simulink library "mylib"  (R2020a)
settings: Solver=VariableStepAuto  StartTime=0.0  StopTime=10.0  RelTol=1e-3
undefined symbols (not defined in the file): d_du_max_pu, dir_to_bus1, dir_to_bus_0L, dir_to_bus_2, dir_to_line1, dir_to_line_0L, dir_to_line_2, du_max_pu, du_ph_max_pu, Fi_0, Fi_T_H, Fi_T_L, Fi_T_M, I0_calc_0L, I0_comp_H, I0_comp_L, I0_comp_M, I0_max_0L, I2_max_2, I_diff1, I_diff2, I_diff3, I_diff4, I_diff5, I_diff_to, I_hight_CT1_G, I_hight_CT2_G, I_low_CT1, I_low_CT2, I_max1, I_max2, I_max3, I_max4, I_max5, I_min_sec_CT1, I_min_sec_CT2, I_unb, Iph_max_0L, Iph_max_2, jmp_in_zone, jmp_in_zone_0L, jmp_in_zone_2, K_dop, max_min1, only_K1_0L, only_K1_2, only_K2_0L, only_K2_2, only_K3_0L, only_K3_2, P_ctl_0, PQ_Fi_ctl_0, Q_ctl_0, S_set_0, set, set1, T_fast, T_I_ctl, T_off, T_on ... (+15)
libraries: $bdroot x184, powerlib_meascontrol x97
(part 5 of 14)

== system mylib/339_i_recalc_ph_v1/RS1 ==
  S : Inport
  R : Inport  Port=2
  12 : Logic  AllPortsSameDT=off  OutDataTypeStr=boolean
  13 : Logic  Operator=NOT  AllPortsSameDT=off  OutDataTypeStr=boolean
  14 : Memory
  15 : Logic  Operator=OR  AllPortsSameDT=off  OutDataTypeStr=boolean
  Q : Outport
  wires:
  13/1 -> 12/2
  S/1 -> 15/2
  R/1 -> 13/1
  15/1 -> 12/1
  12/1 -> Q/1, 14/1
  14/1 -> 15/1

== system mylib/339_i_recalc_ph_v1/RS2 ==
  S : Inport
  R : Inport  Port=2
  12 : Logic  AllPortsSameDT=off  OutDataTypeStr=boolean
  13 : Logic  Operator=NOT  AllPortsSameDT=off  OutDataTypeStr=boolean
  14 : Memory
  15 : Logic  Operator=OR  AllPortsSameDT=off  OutDataTypeStr=boolean
  Q : Outport
  wires:
  13/1 -> 12/2
  S/1 -> 15/2
  R/1 -> 13/1
  15/1 -> 12/1
  12/1 -> Q/1, 14/1
  14/1 -> 15/1

== system mylib/339_i_recalc_ph_v1/ratio_hight1 ==
  hight : Inport
  low : Inport  Port=2
  1 : Switch  Criteria=u2 > Threshold
  15 : RelationalOperator  Operator===  OutDataTypeStr=boolean  RndMeth=Nearest
  16 : Product  Inputs=*/  RndMeth=Zero  SaturateOnIntegerOverflow=on
  17 : RelationalOperator  Operator===  OutDataTypeStr=boolean  RndMeth=Nearest
  18 : Logic  Operator=OR  AllPortsSameDT=off  OutDataTypeStr=boolean
  19 : Constant
  20 : Constant  Value=0
  K : Outport
  wires:
  1/1 -> K/1
  low/1 -> 16/2, 17/1
  15/1 -> 18/1
  19/1 -> 1/1
  17/1 -> 18/2
  16/1 -> 1/3
  20/1 -> 15/2, 17/2
  18/1 -> 1/2
  hight/1 -> 16/1, 15/1

== system mylib/339_i_recalc_ph_v1/ratio_hight18 ==
  hight : Inport
  low : Inport  Port=2
  1 : Switch  Criteria=u2 > Threshold
  15 : RelationalOperator  Operator===  OutDataTypeStr=boolean  RndMeth=Nearest
  16 : Product  Inputs=*/  RndMeth=Zero  SaturateOnIntegerOverflow=on
  17 : RelationalOperator  Operator===  OutDataTypeStr=boolean  RndMeth=Nearest
  18 : Logic  Operator=OR  AllPortsSameDT=off  OutDataTypeStr=boolean
  19 : Constant
  20 : Constant  Value=0
  K : Outport
  wires:
  1/1 -> K/1
  low/1 -> 16/2, 17/1
  15/1 -> 18/1
  19/1 -> 1/1
  17/1 -> 18/2
  16/1 -> 1/3
  20/1 -> 15/2, 17/2
  18/1 -> 1/2
  hight/1 -> 16/1, 15/1

== system mylib/342_u_recalc_ph_v1/K_VT_tr ==
  hight : Inport
  low : Inport  Port=2
  1 : Switch  Criteria=u2 > Threshold
  15 : RelationalOperator  Operator===  OutDataTypeStr=boolean  RndMeth=Nearest
  16 : Product  Inputs=*/  RndMeth=Zero  SaturateOnIntegerOverflow=on
  17 : RelationalOperator  Operator===  OutDataTypeStr=boolean  RndMeth=Nearest
  18 : Logic  Operator=OR  AllPortsSameDT=off  OutDataTypeStr=boolean
  19 : Constant
  20 : Constant  Value=0
  K : Outport
  wires:
  1/1 -> K/1
  low/1 -> 16/2, 17/1
  15/1 -> 18/1
  19/1 -> 1/1
  17/1 -> 18/2
  16/1 -> 1/3
  20/1 -> 15/2, 17/2
  18/1 -> 1/2
  hight/1 -> 16/1, 15/1

== system mylib/342_u_recalc_ph_v1/K_VT_zv ==
  hight : Inport
  low : Inport  Port=2
  1 : Switch  Criteria=u2 > Threshold
  15 : RelationalOperator  Operator===  OutDataTypeStr=boolean  RndMeth=Nearest
  16 : Product  Inputs=*/  RndMeth=Zero  SaturateOnIntegerOverflow=on
  17 : RelationalOperator  Operator===  OutDataTypeStr=boolean  RndMeth=Nearest
  18 : Logic  Operator=OR  AllPortsSameDT=off  OutDataTypeStr=boolean
  19 : Constant
  20 : Constant  Value=0
  K : Outport
  wires:
  1/1 -> K/1
  low/1 -> 16/2, 17/1
  15/1 -> 18/1
  19/1 -> 1/1
  17/1 -> 18/2
  16/1 -> 1/3
  20/1 -> 15/2, 17/2
  18/1 -> 1/2
  hight/1 -> 16/1, 15/1

== system mylib/342_u_recalc_ph_v1/module_Ua_zv ==
  Re : Inport
  Im : Inport  Port=2
  1 : Product  Inputs=**
  2 : Sum
  3 : Product  Inputs=**
  4 : Sqrt  SaturateOnIntegerOverflow=on
  Module : Outport
  wires:
  3/1 -> 2/2
  1/1 -> 2/1
  Im/1 -> 3/1, 3/2
  4/1 -> Module/1
  2/1 -> 4/1
  Re/1 -> 1/2, 1/1

== system mylib/342_u_recalc_ph_v1/module_Uab_zv ==
  Re : Inport
  Im : Inport  Port=2
  1 : Product  Inputs=**
  2 : Sum
  3 : Product  Inputs=**
  4 : Sqrt  SaturateOnIntegerOverflow=on
  Module : Outport
  wires:
  3/1 -> 2/2
  1/1 -> 2/1
  Im/1 -> 3/1, 3/2
  4/1 -> Module/1
  2/1 -> 4/1
  Re/1 -> 1/2, 1/1

== system mylib/342_u_recalc_ph_v1/module_Ub_zv ==
  Re : Inport
  Im : Inport  Port=2
  1 : Product  Inputs=**
  2 : Sum
  3 : Product  Inputs=**
  4 : Sqrt  SaturateOnIntegerOverflow=on
  Module : Outport
  wires:
  3/1 -> 2/2
  1/1 -> 2/1
  Im/1 -> 3/1, 3/2
  4/1 -> Module/1
  2/1 -> 4/1
  Re/1 -> 1/2, 1/1

== system mylib/342_u_recalc_ph_v1/module_Ubc_zv ==
  Re : Inport
  Im : Inport  Port=2
  1 : Product  Inputs=**
  2 : Sum
  3 : Product  Inputs=**
  4 : Sqrt  SaturateOnIntegerOverflow=on
  Module : Outport
  wires:
  3/1 -> 2/2
  1/1 -> 2/1
  Im/1 -> 3/1, 3/2
  4/1 -> Module/1
  2/1 -> 4/1
  Re/1 -> 1/2, 1/1

== system mylib/342_u_recalc_ph_v1/module_Uc_zv ==
  Re : Inport
  Im : Inport  Port=2
  1 : Product  Inputs=**
  2 : Sum
  3 : Product  Inputs=**
  4 : Sqrt  SaturateOnIntegerOverflow=on
  Module : Outport
  wires:
  3/1 -> 2/2
  1/1 -> 2/1
  Im/1 -> 3/1, 3/2
  4/1 -> Module/1
  2/1 -> 4/1
  Re/1 -> 1/2, 1/1

== system mylib/342_u_recalc_ph_v1/module_Uca_zv ==
  Re : Inport
  Im : Inport  Port=2
  1 : Product  Inputs=**
  2 : Sum
  3 : Product  Inputs=**
  4 : Sqrt  SaturateOnIntegerOverflow=on
  Module : Outport
  wires:
  3/1 -> 2/2
  1/1 -> 2/1
  Im/1 -> 3/1, 3/2
  4/1 -> Module/1
  2/1 -> 4/1
  Re/1 -> 1/2, 1/1

== system mylib/342_u_recalc_ph_v1/module_Ufk_tr ==
  Re : Inport
  Im : Inport  Port=2
  1 : Product  Inputs=**
  2 : Sum
  3 : Product  Inputs=**
  4 : Sqrt  SaturateOnIntegerOverflow=on
  Module : Outport
  wires:
  3/1 -> 2/2
  1/1 -> 2/1
  Im/1 -> 3/1, 3/2
  4/1 -> Module/1
  2/1 -> 4/1
  Re/1 -> 1/2, 1/1

== system mylib/342_u_recalc_ph_v1/module_Uhk_tr ==
  Re : Inport
  Im : Inport  Port=2
  1 : Product  Inputs=**
  2 : Sum
  3 : Product  Inputs=**
  4 : Sqrt  SaturateOnIntegerOverflow=on
  Module : Outport
  wires:
  3/1 -> 2/2
  1/1 -> 2/1
  Im/1 -> 3/1, 3/2
  4/1 -> Module/1
  2/1 -> 4/1
  Re/1 -> 1/2, 1/1

== system mylib/342_u_recalc_ph_v1/module_Uhu_tr ==
  Re : Inport
  Im : Inport  Port=2
  1 : Product  Inputs=**
  2 : Sum
  3 : Product  Inputs=**
  4 : Sqrt  SaturateOnIntegerOverflow=on
  Module : Outport
  wires:
  3/1 -> 2/2
  1/1 -> 2/1
  Im/1 -> 3/1, 3/2
  4/1 -> Module/1
  2/1 -> 4/1
  Re/1 -> 1/2, 1/1

== system mylib/342_u_recalc_ph_v1/module_Uuf_tr ==
  Re : Inport
  Im : Inport  Port=2
  1 : Product  Inputs=**
  2 : Sum
  3 : Product  Inputs=**
  4 : Sqrt  SaturateOnIntegerOverflow=on
  Module : Outport
  wires:
  3/1 -> 2/2
  1/1 -> 2/1
  Im/1 -> 3/1, 3/2
  4/1 -> Module/1
  2/1 -> 4/1
  Re/1 -> 1/2, 1/1

== system mylib/Inverse time-delay/ANSI Inverse time-delay ==
  I : Inport
  ANSI_N : Inport  Port=2
  Au_ANSI : Inport  Port=3
  Bu_ANSI : Inport  Port=4
  Cu_ANSI : Inport  Port=5
  Ip : Inport  Port=6
  D : Inport  Port=7
  Constant1 : Constant  Value=6
  Constant2 : Constant  Value=7
  Constant20 : Constant
  Constant21 : Constant  Value=2
  Constant22 : Constant  Value=3
  Constant23 : Constant  Value=4
  Constant25 : Constant  Value=5
  Constant3 : Constant  Value=0
  Constant4 : Constant  Value=8
  Equation ANSI : Subsystem
  Relational Operator{,1..7} (8 alike) : RelationalOperator  Operator===  OutDataTypeStr=boolean  RndMeth=Simplest
  Сoefficient_1 : Subsystem
  Сoefficient_2 : Subsystem
  Сoefficient_3 : Subsystem
  Сoefficient_4 : Subsystem
  Сoefficient_5 : Subsystem
  Сoefficient_6 : Subsystem
  Сoefficient_7 : Subsystem
  Сoefficient_8 User : Subsystem
  td : Outport
  wires:
  Relational Operator/1 -> Сoefficient_1/4(N)
  Constant25/1 -> Relational Operator5/2
  Constant22/1 -> Relational Operator2/2
  Constant3/1 -> Сoefficient_1/3(C_in), Сoefficient_1/2(B_in), Сoefficient_1/1(A_in)
  ANSI_N/1 -> Relational Operator1/1, Relational Operator2/1, Relational Operator7/1, Relational Operator6/1, Relational Operator4/1, Relational Operator5/1, Relational Operator3/1, Relational Operator/1
  Constant23/1 -> Relational Operator3/2
  D/1 -> Equation ANSI/6(D)
  Constant21/1 -> Relational Operator1/2
  Constant20/1 -> Relational Operator/2
  I/1 -> Equation ANSI/2(I)
  Ip/1 -> Equation ANSI/3(Ip)
  Equation ANSI/1(td) -> td/1
  Сoefficient_1/1(A_out) -> Сoefficient_2/1(A_in)
  Сoefficient_1/2(B_out) -> Сoefficient_2/2(B_in)
  Сoefficient_1/3(C_out) -> Сoefficient_2/3(C_in)
  Relational Operator1/1 -> Сoefficient_2/4(N)
  Сoefficient_2/1(A_out) -> Сoefficient_3/1(A_in)
  Сoefficient_2/2(B_out) -> Сoefficient_3/2(B_in)
  Сoefficient_2/3(C_out) -> Сoefficient_3/3(C_in)
  Relational Operator2/1 -> Сoefficient_3/4(N)
  Сoefficient_3/1(A_out) -> Сoefficient_4/1(A_in)
  Сoefficient_3/2(B_out) -> Сoefficient_4/2(B_in)
  Сoefficient_3/3(C_out) -> Сoefficient_4/3(C_in)
  Relational Operator3/1 -> Сoefficient_4/4(N)
  Сoefficient_4/1(A_out) -> Сoefficient_5/1(A_in)
  Сoefficient_4/2(B_out) -> Сoefficient_5/2(B_in)
  Сoefficient_4/3(C_out) -> Сoefficient_5/3(C_in)
  Relational Operator5/1 -> Сoefficient_5/4(N)
  Сoefficient_8 User/1(B_out) -> Equation ANSI/1(B)
  Сoefficient_8 User/2(A_out) -> Equation ANSI/4(A)
  Сoefficient_8 User/3(C_out) -> Equation ANSI/5(C)
  Au_ANSI/1 -> Сoefficient_8 User/5(Au)
  Bu_ANSI/1 -> Сoefficient_8 User/6(Bu)
  Cu_ANSI/1 -> Сoefficient_8 User/7(Cu)
  Сoefficient_5/1(A_out) -> Сoefficient_6/1(A_in)
  Сoefficient_5/2(B_out) -> Сoefficient_6/2(B_in)
  Сoefficient_5/3(C_out) -> Сoefficient_6/3(C_in)
  Constant4/1 -> Relational Operator7/2
  Constant2/1 -> Relational Operator6/2
  Constant1/1 -> Relational Operator4/2
  Relational Operator7/1 -> Сoefficient_8 User/4(N)
  Сoefficient_6/1(A_out) -> Сoefficient_7/1(A_in)
  Сoefficient_6/2(B_out) -> Сoefficient_7/2(B_in)
  Сoefficient_6/3(C_out) -> Сoefficient_7/3(C_in)
  Relational Operator6/1 -> Сoefficient_7/4(N)
  Relational Operator4/1 -> Сoefficient_6/4(N)
  Сoefficient_7/3(C_out) -> Сoefficient_8 User/3(C_in)
  Сoefficient_7/2(B_out) -> Сoefficient_8 User/2(B_in)
  Сoefficient_7/1(A_out) -> Сoefficient_8 User/1(A_in)

== system mylib/Inverse time-delay/ANSI Inverse time-delay inductive disk relay ==
  I : Inport
  ANSI_N_idr : Inport  Port=2
  Au_ANSI_idr : Inport  Port=3
  Bu_ANSI_idr : Inport  Port=4
  Cu_ANSI_idr : Inport  Port=5
  Ip : Inport  Port=6
  D : Inport  Port=7
  Constant1 : Constant  Value=6
  Constant2 : Constant  Value=7
  Constant20 : Constant
  Constant21 : Constant  Value=2
  Constant22 : Constant  Value=3
  Constant23 : Constant  Value=4
  Constant25 : Constant  Value=5
  Constant3 : Constant  Value=0
  Constant4 : Constant  Value=8
  Equation ANSI_idr : Subsystem
  Relational Operator{,1..7} (8 alike) : RelationalOperator  Operator===  OutDataTypeStr=boolean  RndMeth=Simplest
  Сoefficient_1 : Subsystem
  Сoefficient_2 : Subsystem
  Сoefficient_3 : Subsystem
  Сoefficient_4 : Subsystem
  Сoefficient_5 : Subsystem
  Сoefficient_6 : Subsystem
  Сoefficient_7 : Subsystem
  Сoefficient_8 User : Subsystem
  td : Outport
  wires:
  Relational Operator/1 -> Сoefficient_1/4(N)
  Constant25/1 -> Relational Operator5/2
  Constant22/1 -> Relational Operator2/2
  Constant3/1 -> Сoefficient_1/3(C_in), Сoefficient_1/2(B_in), Сoefficient_1/1(A_in)
  ANSI_N_idr/1 -> Relational Operator1/1, Relational Operator2/1, Relational Operator7/1, Relational Operator6/1, Relational Operator4/1, Relational Operator5/1, Relational Operator3/1, Relational Operator/1
  Constant23/1 -> Relational Operator3/2
  D/1 -> Equation ANSI_idr/6(D)
  Constant21/1 -> Relational Operator1/2
  Constant20/1 -> Relational Operator/2
  I/1 -> Equation ANSI_idr/2(I)
  Ip/1 -> Equation ANSI_idr/3(Ip)
  Equation ANSI_idr/1(td) -> td/1
  Сoefficient_1/1(A_out) -> Сoefficient_2/1(A_in)
  Сoefficient_1/2(B_out) -> Сoefficient_2/2(B_in)
  Сoefficient_1/3(C_out) -> Сoefficient_2/3(C_in)
  Relational Operator1/1 -> Сoefficient_2/4(N)
  Сoefficient_2/1(A_out) -> Сoefficient_3/1(A_in)
  Сoefficient_2/2(B_out) -> Сoefficient_3/2(B_in)
  Сoefficient_2/3(C_out) -> Сoefficient_3/3(C_in)
  Relational Operator2/1 -> Сoefficient_3/4(N)
  Сoefficient_3/1(A_out) -> Сoefficient_4/1(A_in)
  Сoefficient_3/2(B_out) -> Сoefficient_4/2(B_in)
  Сoefficient_3/3(C_out) -> Сoefficient_4/3(C_in)
  Relational Operator3/1 -> Сoefficient_4/4(N)
  Сoefficient_4/1(A_out) -> Сoefficient_5/1(A_in)
  Сoefficient_4/2(B_out) -> Сoefficient_5/2(B_in)
  Сoefficient_4/3(C_out) -> Сoefficient_5/3(C_in)
  Relational Operator5/1 -> Сoefficient_5/4(N)
  Сoefficient_8 User/1(B_out) -> Equation ANSI_idr/1(B)
  Сoefficient_8 User/2(A_out) -> Equation ANSI_idr/4(A)
  Сoefficient_8 User/3(C_out) -> Equation ANSI_idr/5(C)
  Au_ANSI_idr/1 -> Сoefficient_8 User/5(Au)
  Bu_ANSI_idr/1 -> Сoefficient_8 User/6(Bu)
  Cu_ANSI_idr/1 -> Сoefficient_8 User/7(Cu)
  Сoefficient_5/1(A_out) -> Сoefficient_6/1(A_in)
  Сoefficient_5/2(B_out) -> Сoefficient_6/2(B_in)
  Сoefficient_5/3(C_out) -> Сoefficient_6/3(C_in)
  Constant4/1 -> Relational Operator7/2
  Constant2/1 -> Relational Operator6/2
  Constant1/1 -> Relational Operator4/2
  Relational Operator7/1 -> Сoefficient_8 User/4(N)
  Сoefficient_6/1(A_out) -> Сoefficient_7/1(A_in)
  Сoefficient_6/2(B_out) -> Сoefficient_7/2(B_in)
  Сoefficient_6/3(C_out) -> Сoefficient_7/3(C_in)
  Relational Operator6/1 -> Сoefficient_7/4(N)
  Relational Operator4/1 -> Сoefficient_6/4(N)
  Сoefficient_7/3(C_out) -> Сoefficient_8 User/3(C_in)
  Сoefficient_7/2(B_out) -> Сoefficient_8 User/2(B_in)
  Сoefficient_7/1(A_out) -> Сoefficient_8 User/1(A_in)

== system mylib/Inverse time-delay/IEC Inverse time-delay ==
  I : Inport
  IEC_N : Inport  Port=2
  ku_IEC : Inport  Port=3
  au_IEC : Inport  Port=4
  Ip : Inport  Port=5
  Tb : Inport  Port=6
  Constant20 : Constant
  Constant21 : Constant  Value=2
  Constant22 : Constant  Value=3
  Constant23 : Constant  Value=4
  Constant25 : Constant  Value=5
  Constant3 : Constant  Value=0
  Equation IEC : Subsystem
  Relational Operator{,1..3,5} (5 alike) : RelationalOperator  Operator===  OutDataTypeStr=boolean  RndMeth=Simplest
  Сoefficient_1 : Subsystem
  Сoefficient_2 : Subsystem
  Сoefficient_3 : Subsystem
  Сoefficient_4 : Subsystem
  Сoefficient_5 User : Subsystem
  td : Outport
  wires:
  Сoefficient_5 User/1(k_out) -> Equation IEC/1(k)
  Сoefficient_1/1(k_out) -> Сoefficient_2/1(k_in)
  Relational Operator/1 -> Сoefficient_1/3(N)
  Relational Operator3/1 -> Сoefficient_4/3(N)
  Constant25/1 -> Relational Operator5/2
  Constant22/1 -> Relational Operator2/2
  Constant3/1 -> Сoefficient_1/2(a_in), Сoefficient_1/1(k_in)
  Relational Operator2/1 -> Сoefficient_3/3(N)
  IEC_N/1 -> Relational Operator1/1, Relational Operator2/1, Relational Operator5/1, Relational Operator3/1, Relational Operator/1
  Constant23/1 -> Relational Operator3/2
  Сoefficient_5 User/2(a_out) -> Equation IEC/3(a)
  Tb/1 -> Equation IEC/5(Tb)
  Relational Operator1/1 -> Сoefficient_2/3(N)
  Constant21/1 -> Relational Operator1/2
  Constant20/1 -> Relational Operator/2
  I/1 -> Equation IEC/2(I)
  Сoefficient_1/2(a_out) -> Сoefficient_2/2(a_in)
  Relational Operator5/1 -> Сoefficient_5 User/3(N)
  Ip/1 -> Equation IEC/4(Ip)
  Equation IEC/1(td) -> td/1
  ku_IEC/1 -> Сoefficient_5 User/4(k_u)
  au_IEC/1 -> Сoefficient_5 User/5(a_u)
  Сoefficient_2/2(a_out) -> Сoefficient_3/2(a_in)
  Сoefficient_2/1(k_out) -> Сoefficient_3/1(k_in)
  Сoefficient_3/1(k_out) -> Сoefficient_4/1(k_in)
  Сoefficient_3/2(a_out) -> Сoefficient_4/2(a_in)
  Сoefficient_4/1(k_out) -> Сoefficient_5 User/1(k)
  Сoefficient_4/2(a_out) -> Сoefficient_5 User/2(a)

== system mylib/Inverse time-delay/IEC Inverse time-delay inductive disk relay ==
  I : Inport
  IEC_N_idr : Inport  Port=2
  ku_IEC_idr : Inport  Port=3
  au_IEC_idr : Inport  Port=4
  Ip : Inport  Port=5
  Tb : Inport  Port=6
  Constant20 : Constant
  Constant21 : Constant  Value=2
  Constant22 : Constant  Value=3
  Constant23 : Constant  Value=4
  Constant25 : Constant  Value=5
  Constant3 : Constant  Value=0
  Equation IEC_idr : Subsystem
  Relational Operator{,1..3,5} (5 alike) : RelationalOperator  Operator===  OutDataTypeStr=boolean  RndMeth=Simplest
  Сoefficient_1 : Subsystem
  Сoefficient_2 : Subsystem
  Сoefficient_3 : Subsystem
  Сoefficient_4 : Subsystem
  Сoefficient_5 User : Subsystem
  td : Outport
  wires:
  Сoefficient_5 User/1(k_out) -> Equation IEC_idr/1(k)
  Сoefficient_1/1(k_out) -> Сoefficient_2/1(k_in)
  Relational Operator/1 -> Сoefficient_1/3(N)
  Relational Operator3/1 -> Сoefficient_4/3(N)
  Constant25/1 -> Relational Operator5/2
  Constant22/1 -> Relational Operator2/2
  Constant3/1 -> Сoefficient_1/2(a_in), Сoefficient_1/1(k_in)
  Сoefficient_4/2(a_out) -> Сoefficient_5 User/2(a)
  Relational Operator2/1 -> Сoefficient_3/3(N)
  IEC_N_idr/1 -> Relational Operator1/1, Relational Operator2/1, Relational Operator5/1, Relational Operator3/1, Relational Operator/1
  Constant23/1 -> Relational Operator3/2
  Сoefficient_4/1(k_out) -> Сoefficient_5 User/1(k)
  Сoefficient_5 User/2(a_out) -> Equation IEC_idr/3(a)
  Tb/1 -> Equation IEC_idr/5(Tb)
  Relational Operator1/1 -> Сoefficient_2/3(N)
  Constant21/1 -> Relational Operator1/2
  Constant20/1 -> Relational Operator/2
  I/1 -> Equation IEC_idr/2(I)
  Сoefficient_1/2(a_out) -> Сoefficient_2/2(a_in)
  Relational Operator5/1 -> Сoefficient_5 User/3(N)
  Ip/1 -> Equation IEC_idr/4(Ip)
  Equation IEC_idr/1(td) -> td/1
  ku_IEC_idr/1 -> Сoefficient_5 User/4(k_u)
  au_IEC_idr/1 -> Сoefficient_5 User/5(a_u)
  Сoefficient_2/2(a_out) -> Сoefficient_3/2(a_in)
  Сoefficient_2/1(k_out) -> Сoefficient_3/1(k_in)
  Сoefficient_3/1(k_out) -> Сoefficient_4/1(k_in)
  Сoefficient_3/2(a_out) -> Сoefficient_4/2(a_in)

== system mylib/derivative/fifo2 ==
  y : Inport
  {1..7} (7 alike) : Memory
  y0 : Outport
  y1 : Outport  Port=2
  y2 : Outport  Port=3
  y3 : Outport  Port=4
  y4 : Outport  Port=5
  y5 : Outport  Port=6
  y6 : Outport  Port=7
  y7 : Outport  Port=8
  wires:
  y/1 -> y0/1, 1/1
  1/1 -> y1/1, 2/1
  2/1 -> 3/1, y2/1
  3/1 -> 4/1, y3/1
  4/1 -> 5/1, y4/1
  5/1 -> 6/1, y5/1
  6/1 -> 7/1, y6/1
  7/1 -> y7/1

== system mylib/relative/fifo1 ==
  y : Inport
  {1..7} (7 alike) : Memory
  y0 : Outport
  y1 : Outport  Port=2
  y2 : Outport  Port=3
  y3 : Outport  Port=4
  y4 : Outport  Port=5
  y5 : Outport  Port=6
  y6 : Outport  Port=7
  y7 : Outport  Port=8
  wires:
  y/1 -> y0/1, 1/1
  1/1 -> y1/1, 2/1
  2/1 -> 3/1, y2/1
  3/1 -> 4/1, y3/1
  4/1 -> 5/1, y4/1
  5/1 -> 6/1, y5/1
  6/1 -> 7/1, y6/1
  7/1 -> y7/1

== system mylib/relative/fifo2 ==
  y : Inport
  {1..7} (7 alike) : Memory
  y0 : Outport
  y1 : Outport  Port=2
  y2 : Outport  Port=3
  y3 : Outport  Port=4
  y4 : Outport  Port=5
  y5 : Outport  Port=6
  y6 : Outport  Port=7
  y7 : Outport  Port=8
  wires:
  y/1 -> y0/1, 1/1
  1/1 -> y1/1, 2/1
  2/1 -> 3/1, y2/1
  3/1 -> 4/1, y3/1
  4/1 -> 5/1, y4/1
  5/1 -> 6/1, y5/1
  6/1 -> 7/1, y6/1
  7/1 -> y7/1

== system mylib/relative/module1 ==
  Re : Inport
  Im : Inport  Port=2
  1 : Product  Inputs=**
  2 : Sum
  3 : Product  Inputs=**
  4 : Sqrt  SaturateOnIntegerOverflow=on
  Module : Outport
  wires:
  3/1 -> 2/2
  1/1 -> 2/1
  Im/1 -> 3/1, 3/2
  4/1 -> Module/1
  2/1 -> 4/1
  Re/1 -> 1/2, 1/1

== system mylib/relative/module2 ==
  Re : Inport
  Im : Inport  Port=2
  1 : Product  Inputs=**
  2 : Sum
  3 : Product  Inputs=**
  4 : Sqrt  SaturateOnIntegerOverflow=on
  Module : Outport
  wires:
  3/1 -> 2/2
  1/1 -> 2/1
  Im/1 -> 3/1, 3/2
  4/1 -> Module/1
  2/1 -> 4/1
  Re/1 -> 1/2, 1/1

== system mylib/relative/module3 ==
  Re : Inport
  Im : Inport  Port=2
  1 : Product  Inputs=**
  2 : Sum
  3 : Product  Inputs=**
  4 : Sqrt  SaturateOnIntegerOverflow=on
  Module : Outport
  wires:
  3/1 -> 2/2
  1/1 -> 2/1
  Im/1 -> 3/1, 3/2
  4/1 -> Module/1
  2/1 -> 4/1
  Re/1 -> 1/2, 1/1

== system mylib/simpcomp/orto_MUL_orto ==
  F1re : Inport
  F1im : Inport  Port=2
  F2re : Inport  Port=3
  F2im : Inport  Port=4
  1 : Sum  Inputs=+-
  {2..5} (4 alike) : Product
  6 : Sum
  Fre : Outport
  Fim : Outport  Port=2
  wires:
  F2re/1 -> 4/2, 2/2
  F1im/1 -> 3/1, 4/1
  F2im/1 -> 3/2, 5/2
  5/1 -> 6/2
  4/1 -> 6/1
  3/1 -> 1/2
  2/1 -> 1/1
  6/1 -> Fim/1
  1/1 -> Fre/1
  F1re/1 -> 2/1, 5/1

== system mylib/simpcomp/orto_MUL_orto1 ==
  F1re : Inport
  F1im : Inport  Port=2
  F2re : Inport  Port=3
  F2im : Inport  Port=4
  1 : Sum  Inputs=+-
  {2..5} (4 alike) : Product
  6 : Sum
  Fre : Outport
  Fim : Outport  Port=2
  wires:
  F2re/1 -> 4/2, 2/2
  F1im/1 -> 3/1, 4/1
  F2im/1 -> 3/2, 5/2
  5/1 -> 6/2
  4/1 -> 6/1
  3/1 -> 1/2
  2/1 -> 1/1
  6/1 -> Fim/1
  1/1 -> Fre/1
  F1re/1 -> 2/1, 5/1

== system mylib/simpcomp/orto_MUL_orto2 ==
  F1re : Inport
  F1im : Inport  Port=2
  F2re : Inport  Port=3
  F2im : Inport  Port=4
  1 : Sum  Inputs=+-
  {2..5} (4 alike) : Product
  6 : Sum
  Fre : Outport
  Fim : Outport  Port=2
  wires:
  F2re/1 -> 4/2, 2/2
  F1im/1 -> 3/1, 4/1
  F2im/1 -> 3/2, 5/2
  5/1 -> 6/2
  4/1 -> 6/1
  3/1 -> 1/2
  2/1 -> 1/1
  6/1 -> Fim/1
  1/1 -> Fre/1
  F1re/1 -> 2/1, 5/1

== system mylib/simpcomp/orto_MUL_orto3 ==
  F1re : Inport
  F1im : Inport  Port=2
  F2re : Inport  Port=3
  F2im : Inport  Port=4
  1 : Sum  Inputs=+-
  {2..5} (4 alike) : Product
  6 : Sum
  Fre : Outport
  Fim : Outport  Port=2
  wires:
  F2re/1 -> 4/2, 2/2
  F1im/1 -> 3/1, 4/1
  F2im/1 -> 3/2, 5/2
  5/1 -> 6/2
  4/1 -> 6/1
  3/1 -> 1/2
  2/1 -> 1/1
  6/1 -> Fim/1
  1/1 -> Fre/1
  F1re/1 -> 2/1, 5/1

== system mylib/st_inverse/Inverse time-delay ==
  I : Inport
  ANSI Inverse time-delay : Subsystem
  ANSI Inverse time-delay inductive disk relay : Subsystem
  Add : Sum
  Constant : Constant  Value=IEC_N
  Constant1 : Constant  Value=ku_IEC
  Constant10 : Constant  Value=Au_ANSI
  Constant11 : Constant  Value=Bu_ANSI
  Constant12 : Constant  Value=Au_ANSI_idr
  Constant13 : Constant  Value=ANSI_N
  Constant14 : Constant  Value=Bu_ANSI_idr
  Constant15 : Constant  Value=ANSI_N_idr
  Constant16 : Constant  Value=Cu_ANSI_idr
  Constant17 : Constant  Value=IDR
  Constant18 : Constant  Value=0
  Constant19 : Constant  Value=0
  Constant2 : Constant  Value=au_IEC
  Constant20 : Constant  Value=Type_ITD
  Constant21 : Constant  Value=Cu_ANSI
  Constant3 : Constant  Value=Tb
  Constant5 : Constant  Value=ku_IEC_idr
  Constant6 : Constant  Value=au_IEC_idr
  Constant7 : Constant  Value=Ip
  Constant8 : Constant  Value=D
  Constant9 : Constant  Value=IEC_N_idr
  IEC Inverse time-delay : Subsystem
  IEC Inverse time-delay inductive disk relay : Subsystem
  Logical Operator : Logic  AllPortsSameDT=off  OutDataTypeStr=boolean
  Logical Operator1 : Logic  AllPortsSameDT=off  OutDataTypeStr=boolean
  Logical Operator4 : Logic  Operator=NOT  AllPortsSameDT=off  OutDataTypeStr=boolean
  Switch1 : Switch  Criteria=u2 > Threshold
  Switch2 : Switch  Criteria=u2 > Threshold
  Switch3 : Switch  Criteria=u2 > Threshold
  tp : Outport
  td : Outport  Port=2
  wires:
  IEC Inverse time-delay/1(td) -> Switch3/1
  Logical Operator4/1 -> Logical Operator1/1
  Constant8/1 -> ANSI Inverse time-delay/7(D), ANSI Inverse time-delay inductive disk relay/7(D)
  Constant6/1 -> IEC Inverse time-delay inductive disk relay/4(au_IEC_idr)
  Constant15/1 -> ANSI Inverse time-delay inductive disk relay/2(ANSI_N_idr)
  Constant16/1 -> ANSI Inverse time-delay inductive disk relay/5(Cu_ANSI_idr)
  Constant12/1 -> ANSI Inverse time-delay inductive disk relay/3(Au_ANSI_idr)
  ANSI Inverse time-delay inductive disk relay/1(td) -> Switch2/1
  Switch2/1 -> Add/2
  Constant/1 -> IEC Inverse time-delay/2(IEC_N)
  Logical Operator1/1 -> Switch2/2
  Constant17/1 -> Logical Operator/2, Logical Operator1/2
  Constant5/1 -> IEC Inverse time-delay inductive disk relay/3(ku_IEC_idr)
  I/1 -> IEC Inverse time-delay inductive disk relay/1(I), ANSI Inverse time-delay inductive disk relay/1(I), ANSI Inverse time-delay/1(I), IEC Inverse time-delay/1(I)
  Constant19/1 -> Switch1/3
  Logical Operator/1 -> Switch1/2
  Switch1/1 -> Add/1
  Constant7/1 -> ANSI Inverse time-delay inductive disk relay/6(Ip), ANSI Inverse time-delay/6(Ip), IEC Inverse time-delay inductive disk relay/5(Ip), IEC Inverse time-delay/5(Ip)
  Switch3/1 -> tp/1
  Constant20/1 -> Logical Operator4/1, Switch3/2, Logical Operator/1
  Constant18/1 -> Switch2/3
  Constant3/1 -> IEC Inverse time-delay inductive disk relay/6(Tb), IEC Inverse time-delay/6(Tb)
  Add/1 -> td/1
  Constant10/1 -> ANSI Inverse time-delay/3(Au_ANSI)
  Constant2/1 -> IEC Inverse time-delay/4(au_IEC)
  IEC Inverse time-delay inductive disk relay/1(td) -> Switch1/1
  Constant11/1 -> ANSI Inverse time-delay/4(Bu_ANSI)
  Constant1/1 -> IEC Inverse time-delay/3(ku_IEC)
  Constant13/1 -> ANSI Inverse time-delay/2(ANSI_N)
  Constant14/1 -> ANSI Inverse time-delay inductive disk relay/4(Bu_ANSI_idr)
  Constant9/1 -> IEC Inverse time-delay inductive disk relay/2(IEC_N_idr)
  Constant21/1 -> ANSI Inverse time-delay/5(Cu_ANSI)
  ANSI Inverse time-delay/1(td) -> Switch3/3

== system mylib/st_inverse/in_1 ==
  jmp_in_zone : Inport
  in : Inport  Port=2
  jmp : Inport  Port=3
  T_reset : Inport  Port=4
  1 : Switch  Criteria=u2 > Threshold
  10 : Logic  AllPortsSameDT=off  OutDataTypeStr=boolean
  11 : Logic  Operator=NOT  AllPortsSameDT=off  OutDataTypeStr=boolean
  12 : Memory
  3 : Logic  AllPortsSameDT=off  OutDataTypeStr=boolean
  Cast To Double : DataTypeConversion  OutDataTypeStr=double
  RS : $bdroot/RS  SystemSampleTime=-1  Latency=0  AutoFrameSizeCalculation=off
  R_TRIG : $bdroot/R_TRIG  SystemSampleTime=-1  Latency=0  AutoFrameSizeCalculation=off
  T1 : powerlib_meascontrol/Logic/On Delay  DelayType=Off delay  delay=T_reset  ic=0  Ts=0
  Variable Transport Delay : VariableTransportDelay  VariableDelayType=Variable transport delay  MaximumDelay=100
  Y : Outport
  wires:
  RS/1 -> 12/1, Y/1
  in/1 -> 11/1, R_TRIG/1, 1/3
  R_TRIG/1 -> 1/1
  jmp_in_zone/1 -> 1/2
  11/1 -> 10/2
  T1/1 -> 3/2
  1/1 -> 3/1
  jmp/1 -> T1/1
  12/1 -> 10/1
  3/1 -> RS/1
  T_reset/1 -> Variable Transport Delay/2
  Variable Transport Delay/1 -> RS/2
  10/1 -> Cast To Double/1
  Cast To Double/1 -> Variable Transport Delay/1

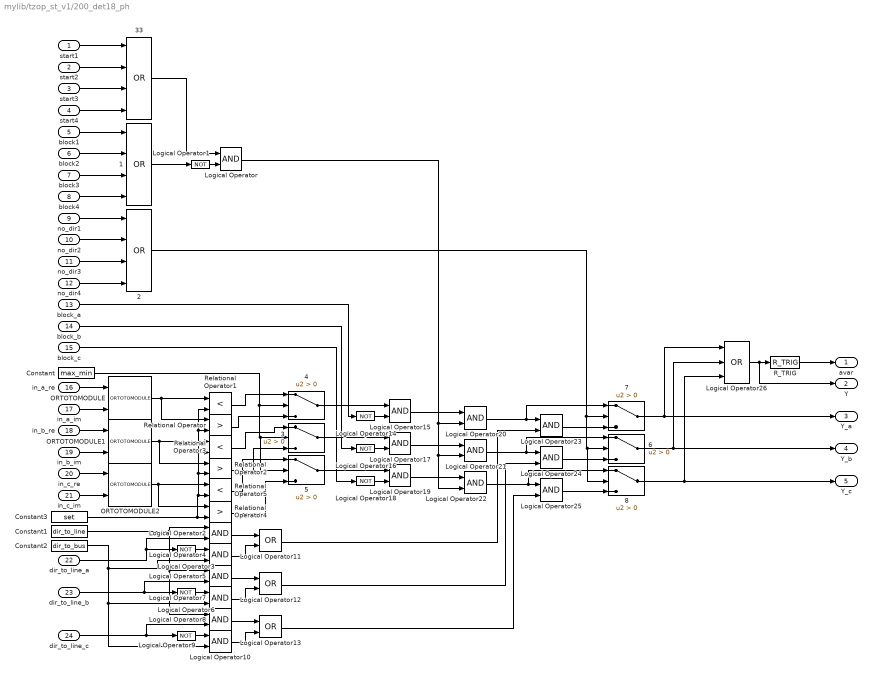
== system mylib/tzop_st_v1/200_det18_ph ==
  start1 : Inport
  start2 : Inport  Port=2
  start3 : Inport  Port=3
  start4 : Inport  Port=4
  block1 : Inport  Port=5
  block2 : Inport  Port=6
  block3 : Inport  Port=7
  block4 : Inport  Port=8
  no_dir1 : Inport  Port=9
  no_dir2 : Inport  Port=10
  no_dir3 : Inport  Port=11
  no_dir4 : Inport  Port=12
  block_a : Inport  Port=13
  block_b : Inport  Port=14
  block_c : Inport  Port=15
  in_a_re : Inport  Port=16
  in_a_im : Inport  Port=17
  in_b_re : Inport  Port=18
  in_b_im : Inport  Port=19
  in_c_re : Inport  Port=20
  in_c_im : Inport  Port=21
  dir_to_line_a : Inport  Port=22
  dir_to_line_b : Inport  Port=23
  dir_to_line_c : Inport  Port=24
  1 : Logic  Operator=OR  Inputs=4  AllPortsSameDT=off  OutDataTypeStr=boolean
  2 : Logic  Operator=OR  Inputs=4  AllPortsSameDT=off  OutDataTypeStr=boolean
  {3..8} (6 alike) : Switch  Criteria=u2 > Threshold
  33 : Logic  Operator=OR  Inputs=4  AllPortsSameDT=off  OutDataTypeStr=boolean
  Constant : Constant  Value=max_min
  Constant1 : Constant  Value=dir_to_line
  Constant2 : Constant  Value=dir_to_bus
  Constant3 : Constant  Value=set
  Logical Operator{,2,4..5,7..8,10,15,17,19..25} (16 alike) : Logic  AllPortsSameDT=off  OutDataTypeStr=boolean
  Logical Operator{1,3,6,9,14,16,18} (7 alike) : Logic  Operator=NOT  AllPortsSameDT=off  OutDataTypeStr=boolean
  Logical Operator11 : Logic  Operator=OR  AllPortsSameDT=off  OutDataTypeStr=boolean
  Logical Operator12 : Logic  Operator=OR  AllPortsSameDT=off  OutDataTypeStr=boolean
  Logical Operator13 : Logic  Operator=OR  AllPortsSameDT=off  OutDataTypeStr=boolean
  Logical Operator26 : Logic  Operator=OR  Inputs=3  AllPortsSameDT=off  OutDataTypeStr=boolean
  ORTOTOMODULE : $bdroot/ORTOTOMODULE  SystemSampleTime=-1  Latency=0  AutoFrameSizeCalculation=off
  ORTOTOMODULE1 : $bdroot/ORTOTOMODULE  SystemSampleTime=-1  Latency=0  AutoFrameSizeCalculation=off
  ORTOTOMODULE2 : $bdroot/ORTOTOMODULE  SystemSampleTime=-1  Latency=0  AutoFrameSizeCalculation=off
  R_TRIG : $bdroot/R_TRIG  SystemSampleTime=-1  Latency=0  AutoFrameSizeCalculation=off
  Relational Operator : RelationalOperator  Operator=>  OutDataTypeStr=boolean  RndMeth=Simplest
  Relational Operator1 : RelationalOperator  Operator=<  OutDataTypeStr=boolean  RndMeth=Simplest
  Relational Operator2 : RelationalOperator  Operator=>  OutDataTypeStr=boolean  RndMeth=Simplest
  Relational Operator3 : RelationalOperator  Operator=<  OutDataTypeStr=boolean  RndMeth=Simplest
  Relational Operator4 : RelationalOperator  Operator=>  OutDataTypeStr=boolean  RndMeth=Simplest
  Relational Operator5 : RelationalOperator  Operator=<  OutDataTypeStr=boolean  RndMeth=Simplest
  avar : Outport
  Y : Outport  Port=2
  Y_a : Outport  Port=3
  Y_b : Outport  Port=4
  Y_c : Outport  Port=5
  wires:
  in_b_re/1 -> ORTOTOMODULE1/1
  R_TRIG/1 -> avar/1
  Logical Operator26/1 -> R_TRIG/1, Y/1
  7/1 -> Logical Operator26/1, Y_a/1
  6/1 -> Logical Operator26/2, Y_b/1
  8/1 -> Logical Operator26/3, Y_c/1
  Logical Operator25/1 -> 8/3
  Logical Operator23/1 -> 7/3
  Logical Operator24/1 -> 6/3
  Logical Operator13/1 -> Logical Operator25/2
  2/1 -> 7/2, 6/2, 8/2
  Logical Operator12/1 -> Logical Operator24/2
  Logical Operator11/1 -> Logical Operator23/2
  Logical Operator22/1 -> Logical Operator25/1, 8/1
  Logical Operator21/1 -> Logical Operator24/1, 6/1
  Logical Operator20/1 -> Logical Operator23/1, 7/1
  Logical Operator/1 -> Logical Operator22/2, Logical Operator21/2, Logical Operator20/2
  Logical Operator19/1 -> Logical Operator22/1
  Logical Operator17/1 -> Logical Operator21/1
  Logical Operator15/1 -> Logical Operator20/1
  block_a/1 -> Logical Operator14/1
  block_b/1 -> Logical Operator16/1
  block_c/1 -> Logical Operator18/1
  5/1 -> Logical Operator19/1
  Logical Operator18/1 -> Logical Operator19/2
  3/1 -> Logical Operator17/1
  Logical Operator16/1 -> Logical Operator17/2
  4/1 -> Logical Operator15/1
  Logical Operator14/1 -> Logical Operator15/2
  Logical Operator10/1 -> Logical Operator13/2
  Logical Operator8/1 -> Logical Operator13/1
  Logical Operator7/1 -> Logical Operator12/2
  Logical Operator5/1 -> Logical Operator12/1
  Logical Operator4/1 -> Logical Operator11/2
  Logical Operator2/1 -> Logical Operator11/1
  Constant2/1 -> Logical Operator10/2, Logical Operator7/2, Logical Operator4/2
  dir_to_line_c/1 -> Logical Operator9/1, Logical Operator8/2
  dir_to_line_b/1 -> Logical Operator6/1, Logical Operator5/2
  Logical Operator9/1 -> Logical Operator10/1
  Logical Operator6/1 -> Logical Operator7/1
  Logical Operator3/1 -> Logical Operator4/1
  dir_to_line_a/1 -> Logical Operator3/1, Logical Operator2/2
  Constant1/1 -> Logical Operator5/1, Logical Operator8/1, Logical Operator2/1
  Relational Operator1/1 -> 4/1
  Constant3/1 -> Relational Operator4/2, Relational Operator5/2, Relational Operator3/2, Relational Operator/2, Relational Operator1/2, Relational Operator2/2
  Relational Operator3/1 -> 3/1
  Relational Operator5/1 -> 5/1
  Relational Operator4/1 -> 5/3
  Relational Operator2/1 -> 3/3
  Relational Operator/1 -> 4/3
  Constant/1 -> 4/2, 3/2, 5/2
  in_c_re/1 -> ORTOTOMODULE2/1
  in_c_im/1 -> ORTOTOMODULE2/2
  ORTOTOMODULE2/1 -> Relational Operator4/1, Relational Operator5/1
  in_b_im/1 -> ORTOTOMODULE1/2
  ORTOTOMODULE1/1 -> Relational Operator3/1, Relational Operator2/1
  ORTOTOMODULE/1 -> Relational Operator/1, Relational Operator1/1
  in_a_re/1 -> ORTOTOMODULE/1
  in_a_im/1 -> ORTOTOMODULE/2
  33/1 -> Logical Operator/1
  1/1 -> Logical Operator1/1
  Logical Operator1/1 -> Logical Operator/2
  no_dir4/1 -> 2/4
  no_dir3/1 -> 2/3
  no_dir2/1 -> 2/2
  no_dir1/1 -> 2/1
  block4/1 -> 1/4
  block3/1 -> 1/3
  block2/1 -> 1/2
  block1/1 -> 1/1
  start2/1 -> 33/2
  start3/1 -> 33/3
  start4/1 -> 33/4
  start1/1 -> 33/1

== system mylib/tzop_st_v1/218_det18 ==
  start1 : Inport
  start2 : Inport  Port=2
  start3 : Inport  Port=3
  start4 : Inport  Port=4
  block1 : Inport  Port=5
  block2 : Inport  Port=6
  block3 : Inport  Port=7
  block4 : Inport  Port=8
  no_dir1 : Inport  Port=9
  no_dir2 : Inport  Port=10
  no_dir3 : Inport  Port=11
  no_dir4 : Inport  Port=12
  in_re : Inport  Port=13
  in_im : Inport  Port=14
  dir_to_line : Inport  Port=15
  1 : Logic  Operator=OR  Inputs=4  AllPortsSameDT=off  OutDataTypeStr=boolean
  2 : Logic  Operator=OR  Inputs=4  AllPortsSameDT=off  OutDataTypeStr=boolean
  33 : Logic  Operator=OR  Inputs=4  AllPortsSameDT=off  OutDataTypeStr=boolean
  4 : Switch  Criteria=u2 > Threshold
  7 : Switch  Criteria=u2 > Threshold
  Constant : Constant  Value=max_min
  Constant1 : Constant  Value=dir_to_line
  Constant2 : Constant  Value=dir_to_bus
  Constant3 : Constant  Value=set
  Logical Operator{,2,4,20,23} (5 alike) : Logic  AllPortsSameDT=off  OutDataTypeStr=boolean
  Logical Operator1 : Logic  Operator=NOT  AllPortsSameDT=off  OutDataTypeStr=boolean
  Logical Operator11 : Logic  Operator=OR  AllPortsSameDT=off  OutDataTypeStr=boolean
  Logical Operator3 : Logic  Operator=NOT  AllPortsSameDT=off  OutDataTypeStr=boolean
  ORTOTOMODULE : $bdroot/ORTOTOMODULE  SystemSampleTime=-1  Latency=0  AutoFrameSizeCalculation=off
  R_TRIG : $bdroot/R_TRIG  SystemSampleTime=-1  Latency=0  AutoFrameSizeCalculation=off
  Relational Operator : RelationalOperator  Operator=>  OutDataTypeStr=boolean  RndMeth=Simplest
  Relational Operator1 : RelationalOperator  Operator=<  OutDataTypeStr=boolean  RndMeth=Simplest
  avar : Outport
  Y : Outport  Port=2
  wires:
  R_TRIG/1 -> avar/1
  7/1 -> R_TRIG/1, Y/1
  Logical Operator23/1 -> 7/3
  2/1 -> 7/2
  Logical Operator11/1 -> Logical Operator23/2
  Logical Operator20/1 -> Logical Operator23/1, 7/1
  Logical Operator/1 -> Logical Operator20/2
  4/1 -> Logical Operator20/1
  Logical Operator4/1 -> Logical Operator11/2
  Logical Operator2/1 -> Logical Operator11/1
  Constant2/1 -> Logical Operator4/1
  Logical Operator3/1 -> Logical Operator4/2
  dir_to_line/1 -> Logical Operator3/1, Logical Operator2/2
  Constant1/1 -> Logical Operator2/1
  Relational Operator1/1 -> 4/1
  Constant3/1 -> Relational Operator/2, Relational Operator1/2
  Relational Operator/1 -> 4/3
  Constant/1 -> 4/2
  ORTOTOMODULE/1 -> Relational Operator/1, Relational Operator1/1
  in_re/1 -> ORTOTOMODULE/1
  in_im/1 -> ORTOTOMODULE/2
  33/1 -> Logical Operator/1
  1/1 -> Logical Operator1/1
  Logical Operator1/1 -> Logical Operator/2
  no_dir4/1 -> 2/4
  no_dir3/1 -> 2/3
  no_dir2/1 -> 2/2
  no_dir1/1 -> 2/1
  block4/1 -> 1/4
  block3/1 -> 1/3
  block2/1 -> 1/2
  block1/1 -> 1/1
  start2/1 -> 33/2
  start3/1 -> 33/3
  start4/1 -> 33/4
  start1/1 -> 33/1

== system mylib/tzop_st_v1/230_st18_ph ==
  fast1_time : Inport
  fast2_time : Inport  Port=2
  fast1_zero : Inport  Port=3
  fast2_zero : Inport  Port=4
  block1 : Inport  Port=5
  block2 : Inport  Port=6
  block3 : Inport  Port=7
  block4 : Inport  Port=8
  in_a : Inport  Port=9
  in_b : Inport  Port=10
  in_c : Inport  Port=11
  alt_in_a : Inport  Port=12
  alt_in_b : Inport  Port=13
  alt_in_c : Inport  Port=14
  jmp_a : Inport  Port=15
  jmp_b : Inport  Port=16
  jmp_c : Inport  Port=17
  1 : Logic  Operator=OR  Inputs=4  AllPortsSameDT=off  OutDataTypeStr=boolean
  Constant1 : Constant  Value=only_K2
  Constant2 : Constant  Value=only_K3
  Constant3 : Constant  Value=only_K1
  Constant4 : Constant  Value=jmp_in_zone
  Logical Operator1 : Logic  Operator=OR  Inputs=3  AllPortsSameDT=off  OutDataTypeStr=boolean
  Logical Operator10 : Logic  Inputs=3  AllPortsSameDT=off  OutDataTypeStr=boolean
  Logical Operator{2,4,6,11..13} (6 alike) : Logic  AllPortsSameDT=off  OutDataTypeStr=boolean
  Logical Operator{14,16..17,27..28} (5 alike) : Logic  Operator=OR  AllPortsSameDT=off  OutDataTypeStr=boolean
  Logical Operator26 : Logic  Operator=OR  Inputs=3  AllPortsSameDT=off  OutDataTypeStr=boolean
  Logical Operator3 : Logic  Operator=NOT  AllPortsSameDT=off  OutDataTypeStr=boolean
  Logical Operator5 : Logic  Operator=NOT  AllPortsSameDT=off  OutDataTypeStr=boolean
  Logical Operator7 : Logic  Operator=NOT  AllPortsSameDT=off  OutDataTypeStr=boolean
  Logical Operator8 : Logic  Inputs=3  AllPortsSameDT=off  OutDataTypeStr=boolean
  Logical Operator9 : Logic  Inputs=3  AllPortsSameDT=off  OutDataTypeStr=boolean
  R_TRIG : $bdroot/R_TRIG  SystemSampleTime=-1  Latency=0  AutoFrameSizeCalculation=off
  Subsystem : Subsystem  mask{time=[T_fast, T_st]}
      mask prompts: time "time [T_fast, T_st]"
  in_1 : Subsystem  mask{in_jmp=[T_reset]}
      mask prompts: in_jmp "in_jmp[T_reset]"
  in_2 : Subsystem  mask{in_jmp=[T_reset]}
      mask prompts: in_jmp "in_jmp[T_reset]"
  in_3 : Subsystem  mask{in_jmp=[T_reset]}
      mask prompts: in_jmp "in_jmp[T_reset]"
  k_type : Subsystem
  out_a : $bdroot/out3  out=[T_out]
  out_b : $bdroot/out3  out=[T_out]
  out_c : $bdroot/out3  out=[T_out]
  avar : Outport
  Y : Outport  Port=2
  Y_a : Outport  Port=3
  Y_b : Outport  Port=4
  Y_c : Outport  Port=5
  fast : Outport  Port=6
  fast_a : Outport  Port=7
  fast_b : Outport  Port=8
  fast_c : Outport  Port=9
  wires:
  Logical Operator1/1 -> fast/1
  Logical Operator28/1 -> Subsystem/2(T_fast_zero)
  Logical Operator27/1 -> Subsystem/1(T_fast_time)
  alt_in_c/1 -> Logical Operator17/2
  alt_in_b/1 -> Logical Operator16/2
  alt_in_a/1 -> Logical Operator14/2
  Logical Operator14/1 -> Subsystem/3("In1 ")
  Logical Operator16/1 -> Subsystem/4("In2 ")
  Logical Operator17/1 -> Subsystem/5("In3 ")
  Logical Operator13/1 -> Logical Operator17/1
  Logical Operator12/1 -> Logical Operator16/1
  Logical Operator11/1 -> Logical Operator14/1
  k_type/1(out) -> Logical Operator11/1, Logical Operator13/1, Logical Operator12/1, Logical Operator8/3, Logical Operator9/3, Logical Operator10/3
  Constant2/1 -> k_type/6(only_K3)
  Constant1/1 -> k_type/5(only_K2)
  Constant3/1 -> k_type/4(only_K1)
  Logical Operator6/1 -> k_type/3(In_ c), Logical Operator13/2, fast_c/1, Logical Operator1/3
  Logical Operator4/1 -> k_type/2(In_b), Logical Operator12/2, fast_b/1, Logical Operator1/2
  Logical Operator2/1 -> k_type/1(In_a), Logical Operator11/2, fast_a/1, Logical Operator1/1
  Subsystem/1(Out1) -> Logical Operator8/2
  Subsystem/2(Out2) -> Logical Operator9/2
  Subsystem/3(Out3) -> Logical Operator10/2
  Logical Operator10/1 -> out_c/1
  Logical Operator9/1 -> out_b/1
  Logical Operator8/1 -> out_a/1
  out_c/1 -> Y_c/1, Logical Operator26/3  "Y_c"
  out_b/1 -> Y_b/1, Logical Operator26/2  "Y_c"
  out_a/1 -> Y_a/1, Logical Operator26/1  "Y_c"
  1/1 -> Logical Operator3/1, Logical Operator5/1, Logical Operator7/1
  in_3/1(Y) -> Logical Operator6/2  "Yc"
  Logical Operator7/1 -> Logical Operator6/1
  in_2/1(Y) -> Logical Operator4/2  "Yb"
  Logical Operator5/1 -> Logical Operator4/1
  in_1/1(Y) -> Logical Operator2/2  "Ya"
  Logical Operator3/1 -> Logical Operator2/1
  jmp_c/1 -> in_3/3(jmp)
  jmp_b/1 -> in_2/3(jmp)
  jmp_a/1 -> in_1/3(jmp)
  Constant4/1 -> in_1/1(jmp_in_zone), in_2/1(jmp_in_zone), in_3/1(jmp_in_zone)
  in_b/1 -> Logical Operator9/1, in_2/2(in)
  R_TRIG/1 -> avar/1
  Logical Operator26/1 -> R_TRIG/1, Y/1
  in_c/1 -> Logical Operator10/1, in_3/2(in)
  in_a/1 -> Logical Operator8/1, in_1/2(in)
  block4/1 -> 1/4
  block3/1 -> 1/3
  block2/1 -> 1/2
  block1/1 -> 1/1
  fast2_time/1 -> Logical Operator27/2
  fast1_zero/1 -> Logical Operator28/1
  fast2_zero/1 -> Logical Operator28/2
  fast1_time/1 -> Logical Operator27/1

== system mylib/231_u_block_v1/U_ctl_calc19/d_da_db_abs ==
  Re : Inport
  Im : Inport  Port=2
  1 : Product  Inputs=**
  2 : Sum
  3 : Product  Inputs=**
  4 : Sqrt  SaturateOnIntegerOverflow=on
  Module : Outport
  wires:
  3/1 -> 2/2
  1/1 -> 2/1
  Im/1 -> 3/2, 3/1
  4/1 -> Module/1
  2/1 -> 4/1
  Re/1 -> 1/2, 1/1

== system mylib/231_u_block_v1/U_ctl_calc19/d_db_dc_abs ==
  Re : Inport
  Im : Inport  Port=2
  1 : Product  Inputs=**
  2 : Sum
  3 : Product  Inputs=**
  4 : Sqrt  SaturateOnIntegerOverflow=on
  Module : Outport
  wires:
  3/1 -> 2/2
  1/1 -> 2/1
  Im/1 -> 3/1, 3/2
  4/1 -> Module/1
  2/1 -> 4/1
  Re/1 -> 1/2, 1/1

== system mylib/231_u_block_v1/U_ctl_calc19/d_dc_da_abs ==
  Re : Inport
  Im : Inport  Port=2
  1 : Product  Inputs=**
  2 : Sum
  3 : Product  Inputs=**
  4 : Sqrt  SaturateOnIntegerOverflow=on
  Module : Outport
  wires:
  3/1 -> 2/2
  1/1 -> 2/1
  Im/1 -> 3/1, 3/2
  4/1 -> Module/1
  2/1 -> 4/1
  Re/1 -> 1/2, 1/1

== system mylib/231_u_block_v1/U_ctl_calc19/da ==
  Re : Inport
  Im : Inport  Port=2
  1 : Product  Inputs=**
  2 : Sum
  3 : Product  Inputs=**
  4 : Sqrt  SaturateOnIntegerOverflow=on
  Module : Outport
  wires:
  3/1 -> 2/2
  1/1 -> 2/1
  Im/1 -> 3/1, 3/2
  4/1 -> Module/1
  2/1 -> 4/1
  Re/1 -> 1/2, 1/1

== system mylib/231_u_block_v1/U_ctl_calc19/db ==
  Re : Inport
  Im : Inport  Port=2
  1 : Product  Inputs=**
  2 : Sum
  3 : Product  Inputs=**
  4 : Sqrt  SaturateOnIntegerOverflow=on
  Module : Outport
  wires:
  3/1 -> 2/2
  1/1 -> 2/1
  Im/1 -> 3/1, 3/2
  4/1 -> Module/1
  2/1 -> 4/1
  Re/1 -> 1/2, 1/1

== system mylib/231_u_block_v1/U_ctl_calc19/dc ==
  Re : Inport
  Im : Inport  Port=2
  1 : Product  Inputs=**
  2 : Sum
  3 : Product  Inputs=**
  4 : Sqrt  SaturateOnIntegerOverflow=on
  Module : Outport
  wires:
  3/1 -> 2/2
  1/1 -> 2/1
  Im/1 -> 3/1, 3/2
  4/1 -> Module/1
  2/1 -> 4/1
  Re/1 -> 1/2, 1/1

== system mylib/231_u_block_v1/U_ctl_calc19/module_Ua_tr ==
  Re : Inport
  Im : Inport  Port=2
  1 : Product  Inputs=**
  2 : Sum
  3 : Product  Inputs=**
  4 : Sqrt  SaturateOnIntegerOverflow=on
  Module : Outport
  wires:
  3/1 -> 2/2
  1/1 -> 2/1
  Im/1 -> 3/1, 3/2
  4/1 -> Module/1
  2/1 -> 4/1
  Re/1 -> 1/2, 1/1

== system mylib/231_u_block_v1/U_ctl_calc19/module_Ua_zv ==
  Re : Inport
  Im : Inport  Port=2
  1 : Product  Inputs=**
  2 : Sum
  3 : Product  Inputs=**
  4 : Sqrt  SaturateOnIntegerOverflow=on
  Module : Outport
  wires:
  3/1 -> 2/2
  1/1 -> 2/1
  Im/1 -> 3/1, 3/2
  4/1 -> Module/1
  2/1 -> 4/1
  Re/1 -> 1/2, 1/1

== system mylib/231_u_block_v1/U_ctl_calc19/module_Ua_zv1 ==
  Re : Inport
  Im : Inport  Port=2
  1 : Product  Inputs=**
  2 : Sum
  3 : Product  Inputs=**
  4 : Sqrt  SaturateOnIntegerOverflow=on
  Module : Outport
  wires:
  3/1 -> 2/2
  1/1 -> 2/1
  Im/1 -> 3/1, 3/2
  4/1 -> Module/1
  2/1 -> 4/1
  Re/1 -> 1/2, 1/1

== system mylib/231_u_block_v1/U_ctl_calc19/module_Ub_tr ==
  Re : Inport
  Im : Inport  Port=2
  1 : Product  Inputs=**
  2 : Sum
  3 : Product  Inputs=**
  4 : Sqrt  SaturateOnIntegerOverflow=on
  Module : Outport
  wires:
  3/1 -> 2/2
  1/1 -> 2/1
  Im/1 -> 3/1, 3/2
  4/1 -> Module/1
  2/1 -> 4/1
  Re/1 -> 1/2, 1/1

== system mylib/231_u_block_v1/U_ctl_calc19/module_Uc_tr ==
  Re : Inport
  Im : Inport  Port=2
  1 : Product  Inputs=**
  2 : Sum
  3 : Product  Inputs=**
  4 : Sqrt  SaturateOnIntegerOverflow=on
  Module : Outport
  wires:
  3/1 -> 2/2
  1/1 -> 2/1
  Im/1 -> 3/1, 3/2
  4/1 -> Module/1
  2/1 -> 4/1
  Re/1 -> 1/2, 1/1

== system mylib/231_u_block_v1/U_ctl_calc19/module_Uc_zv ==
  Re : Inport
  Im : Inport  Port=2
  1 : Product  Inputs=**
  2 : Sum
  3 : Product  Inputs=**
  4 : Sqrt  SaturateOnIntegerOverflow=on
  Module : Outport
  wires:
  3/1 -> 2/2
  1/1 -> 2/1
  Im/1 -> 3/1, 3/2
  4/1 -> Module/1
  2/1 -> 4/1
  Re/1 -> 1/2, 1/1

== system mylib/231_u_block_v1/U_ctl_logic19/RS ==
  S : Inport
  R : Inport  Port=2
  12 : Logic  AllPortsSameDT=off  OutDataTypeStr=boolean
  13 : Logic  Operator=NOT  AllPortsSameDT=off  OutDataTypeStr=boolean
  14 : Memory
  15 : Logic  Operator=OR  AllPortsSameDT=off  OutDataTypeStr=boolean
  Q : Outport
  wires:
  13/1 -> 12/2
  S/1 -> 15/2
  R/1 -> 13/1
  15/1 -> 12/1
  12/1 -> Q/1, 14/1
  14/1 -> 15/1

== system mylib/231_u_block_v1/U_ctl_logic19/RS1 ==
  S : Inport
  R : Inport  Port=2
  12 : Logic  AllPortsSameDT=off  OutDataTypeStr=boolean
  13 : Logic  Operator=NOT  AllPortsSameDT=off  OutDataTypeStr=boolean
  14 : Memory
  15 : Logic  Operator=OR  AllPortsSameDT=off  OutDataTypeStr=boolean
  Q : Outport
  wires:
  13/1 -> 12/2
  S/1 -> 15/2
  R/1 -> 13/1
  15/1 -> 12/1
  12/1 -> Q/1, 14/1
  14/1 -> 15/1

== system mylib/231_u_block_v1/U_ctl_logic19/r1 ==
  CLK : Inport
  26 : Logic  AllPortsSameDT=off  OutDataTypeStr=boolean
  27 : Logic  Operator=NOT  AllPortsSameDT=off  OutDataTypeStr=boolean
  Memory : Memory
  Q : Outport
  wires:
  27/1 -> 26/2
  Memory/1 -> 27/1
  CLK/1 -> Memory/1, 26/1
  26/1 -> Q/1

== system mylib/231_u_block_v1/U_ctl_logic19/r2 ==
  CLK : Inport
  26 : Logic  AllPortsSameDT=off  OutDataTypeStr=boolean
  27 : Logic  Operator=NOT  AllPortsSameDT=off  OutDataTypeStr=boolean
  Memory : Memory
  Q : Outport
  wires:
  27/1 -> 26/2
  Memory/1 -> 27/1
  CLK/1 -> Memory/1, 26/1
  26/1 -> Q/1

== system mylib/231_u_block_v1/U_ctl_logic19/r3 ==
  CLK : Inport
  26 : Logic  AllPortsSameDT=off  OutDataTypeStr=boolean
  27 : Logic  Operator=NOT  AllPortsSameDT=off  OutDataTypeStr=boolean
  Memory : Memory
  Q : Outport
  wires:
  27/1 -> 26/2
  Memory/1 -> 27/1
  CLK/1 -> Memory/1, 26/1
  26/1 -> Q/1

== system mylib/262_tnznp_line_st_v1/230_st18_ph/Subsystem ==
  T_fast_time : Inport
  T_fast_zero : Inport  Port=2
  "In1 " : Inport  Port=3
  "In2 " : Inport  Port=4
  "In3 " : Inport  Port=5
  {1..5,7} (6 alike) : Switch  Criteria=u2 > Threshold
  T1 : powerlib_meascontrol/Logic/On Delay  DelayType=On delay  delay=T_st  ic=1  Ts=0
  T2 : powerlib_meascontrol/Logic/On Delay  DelayType=On delay  delay=T_st  ic=1  Ts=0
  T3 : powerlib_meascontrol/Logic/On Delay  DelayType=On delay  delay=T_st  ic=1  Ts=0
  T4 : powerlib_meascontrol/Logic/On Delay  DelayType=On delay  delay=T_fast  ic=1  Ts=0
  T5 : powerlib_meascontrol/Logic/On Delay  DelayType=On delay  delay=T_fast  ic=1  Ts=0
  T6 : powerlib_meascontrol/Logic/On Delay  DelayType=On delay  delay=T_fast  ic=1  Ts=0
  T7 : powerlib_meascontrol/Logic/On Delay  DelayType=Off delay  delay=T_fast  ic=1  Ts=0
  Out1 : Outport
  Out2 : Outport  Port=2
  Out3 : Outport  Port=3
  wires:
  4/1 -> Out3/1
  3/1 -> Out2/1
  5/1 -> Out1/1
  2/1 -> 4/3
  1/1 -> 3/3
  7/1 -> 5/3
  T_fast_zero/1 -> 4/2, 3/2, 5/2
  T2/1 -> 2/3
  T1/1 -> 1/3
  T3/1 -> 7/3
  T6/1 -> 7/1
  T5/1 -> 1/1
  T4/1 -> 2/1
  T_fast_time/1 -> T7/1
  T7/1 -> 7/2, 1/2, 2/2
  "In1 "/1 -> T6/1, T3/1, 5/1
  "In2 "/1 -> T1/1, T5/1, 3/1
  "In3 "/1 -> 4/1, T2/1, T4/1

== system mylib/262_tnznp_line_st_v1/230_st18_ph/in_1 ==
  jmp_in_zone : Inport
  in : Inport  Port=2
  jmp : Inport  Port=3
  1 : Switch  Criteria=u2 > Threshold
  10 : Logic  AllPortsSameDT=off  OutDataTypeStr=boolean
  11 : Logic  Operator=NOT  AllPortsSameDT=off  OutDataTypeStr=boolean
  12 : Memory
  3 : Logic  AllPortsSameDT=off  OutDataTypeStr=boolean
  RS : $bdroot/RS  SystemSampleTime=-1  Latency=0  AutoFrameSizeCalculation=off
  R_TRIG : $bdroot/R_TRIG  SystemSampleTime=-1  Latency=0  AutoFrameSizeCalculation=off
  T1 : powerlib_meascontrol/Logic/On Delay  DelayType=Off delay  delay=T_reset  ic=1  Ts=0
  T2 : powerlib_meascontrol/Logic/On Delay  DelayType=On delay  delay=T_reset  ic=1  Ts=0
  Y : Outport
  wires:
  3/1 -> RS/1
  T2/1 -> RS/2
  12/1 -> 10/1
  jmp/1 -> T1/1
  1/1 -> 3/1
  T1/1 -> 3/2
  10/1 -> T2/1
  11/1 -> 10/2
  jmp_in_zone/1 -> 1/2
  R_TRIG/1 -> 1/1
  in/1 -> 1/3, R_TRIG/1, 11/1
  RS/1 -> Y/1, 12/1

== system mylib/262_tnznp_line_st_v1/230_st18_ph/in_2 ==
  jmp_in_zone : Inport
  in : Inport  Port=2
  jmp : Inport  Port=3
  1 : Switch  Criteria=u2 > Threshold
  10 : Logic  AllPortsSameDT=off  OutDataTypeStr=boolean
  11 : Logic  Operator=NOT  AllPortsSameDT=off  OutDataTypeStr=boolean
  12 : Memory
  3 : Logic  AllPortsSameDT=off  OutDataTypeStr=boolean
  RS : $bdroot/RS  SystemSampleTime=-1  Latency=0  AutoFrameSizeCalculation=off
  R_TRIG : $bdroot/R_TRIG  SystemSampleTime=-1  Latency=0  AutoFrameSizeCalculation=off
  T1 : powerlib_meascontrol/Logic/On Delay  DelayType=Off delay  delay=T_reset  ic=1  Ts=0
  T2 : powerlib_meascontrol/Logic/On Delay  DelayType=On delay  delay=T_reset  ic=1  Ts=0
  Y : Outport
  wires:
  3/1 -> RS/1
  T2/1 -> RS/2
  12/1 -> 10/1
  jmp/1 -> T1/1
  1/1 -> 3/1
  T1/1 -> 3/2
  10/1 -> T2/1
  11/1 -> 10/2
  jmp_in_zone/1 -> 1/2
  R_TRIG/1 -> 1/1
  in/1 -> 1/3, R_TRIG/1, 11/1
  RS/1 -> Y/1, 12/1

== system mylib/262_tnznp_line_st_v1/230_st18_ph/in_3 ==
  jmp_in_zone : Inport
  in : Inport  Port=2
  jmp : Inport  Port=3
  1 : Switch  Criteria=u2 > Threshold
  10 : Logic  AllPortsSameDT=off  OutDataTypeStr=boolean
  11 : Logic  Operator=NOT  AllPortsSameDT=off  OutDataTypeStr=boolean
  12 : Memory
  3 : Logic  AllPortsSameDT=off  OutDataTypeStr=boolean
  RS : $bdroot/RS  SystemSampleTime=-1  Latency=0  AutoFrameSizeCalculation=off
  R_TRIG : $bdroot/R_TRIG  SystemSampleTime=-1  Latency=0  AutoFrameSizeCalculation=off
  T1 : powerlib_meascontrol/Logic/On Delay  DelayType=Off delay  delay=T_reset  ic=1  Ts=0
  T2 : powerlib_meascontrol/Logic/On Delay  DelayType=On delay  delay=T_reset  ic=1  Ts=0
  Y : Outport
  wires:
  3/1 -> RS/1
  T2/1 -> RS/2
  12/1 -> 10/1
  jmp/1 -> T1/1
  1/1 -> 3/1
  T1/1 -> 3/2
  10/1 -> T2/1
  11/1 -> 10/2
  jmp_in_zone/1 -> 1/2
  R_TRIG/1 -> 1/1
  in/1 -> 1/3, R_TRIG/1, 11/1
  RS/1 -> Y/1, 12/1
